simulink model "QueuingSys"  (R2019a)
settings: Solver=VariableStepAuto  StartTime=0.0  StopTime=100  RelTol=1e-3  EnableMultiTasking=on
undefined symbols (not defined in the file or in its folder): m, n
(part 4 of 5)

== system QueuingSys/Distro/MMPPArrivalTime57 ==
  MMPPArrivalTime : TriggerPort  TriggerType=function-call  IsSimulinkFunction=on  FunctionName=MMPPArrivalTime57  VariantControl=Variant
  Constant : Constant  Value=[0.495890558927082 0.224465538335651 0.279643902737266;0.534632777235722 0.436142153474273 0.0292250692900047;0.092615054756791 0.5282924947216 0.379092450521609]  SampleTime=-1
  D : Memory  InitialCondition=[0.615571878010216;0.243014654438024]  InheritSampleTime=on
  MMPP : MATLAB Function  TreatAsAtomicUnit=on
  Scope : Scope
  Scope1 : Scope
  T : Memory  InitialCondition=[0 0.156984443601208]  InheritSampleTime=on
  Uniform Random Number : UniformRandomNumber  Minimum=0  Seed=randi(5000)
  X : Memory  InitialCondition=2  InheritSampleTime=on
  t : ArgOut  DisableCoverage=on  ArgumentName=t
  wires:
  MMPP/5(lambda) -> Scope1/1
  D/1 -> MMPP/3("D ")
  MMPP/3(D) -> D/1
  Uniform Random Number/1 -> MMPP/5(rn)
  Constant/1 -> MMPP/4(M)
  MMPP/1(x) -> X/1
  MMPP/4(t) -> Scope/1, t/1
  MMPP/2(T) -> T/1
  T/1 -> MMPP/2("T ")
  X/1 -> MMPP/1("x ")

== system QueuingSys/Distro/MMPPArrivalTime58 ==
  MMPPArrivalTime : TriggerPort  TriggerType=function-call  IsSimulinkFunction=on  FunctionName=MMPPArrivalTime58  VariantControl=Variant
  Constant : Constant  Value=[0.117464299599952 0.152250567651033 0.121837267495483 0.159738037776046 0.149409502151923 0.125667086953631 0.173633238371933;0.148836709986002 0.0654920343032583 0.211732490033451 0.0881549893916536 0.208284652862022 0.1607543990228 0.116744724400813;0.197470470038891 0.0885266634647723 0.271156507153938 0.0722093849692539 0.0815411153869947 0.0614322791512611 0.227663579834889;0.1864274555943 0.0103838777427165 0.409677435278208 0.122348195829911 0.0518869784402073 0.187281746714561 0.0319943104000951;0.126572465826877 0.141130417950956 0.0378088808905448 0.0689503315505311 0.0237192420773743 0.137680845625693 0.464137816078024;0.175039845353253 0.101735916497746 0.151094631354237 0.0556980729938636 0.0793353789695721 0.239650762795073 0.197445392036255;0.164973290584489 0.169364680581661 0.0117698334218001 0.217271387849719 0.171379794259574 0.197448646262573 0.0677923670401836]  SampleTime=-1
  D : Memory  InitialCondition=[0.478618395085393;0.871374928352472]  InheritSampleTime=on
  MMPP : MATLAB Function  TreatAsAtomicUnit=on
  Scope : Scope
  Scope1 : Scope
  T : Memory  InitialCondition=[0 1.559364915483]  InheritSampleTime=on
  Uniform Random Number : UniformRandomNumber  Minimum=0  Seed=randi(5000)
  X : Memory  InitialCondition=6  InheritSampleTime=on
  t : ArgOut  DisableCoverage=on  ArgumentName=t
  wires:
  MMPP/5(lambda) -> Scope1/1
  D/1 -> MMPP/3("D ")
  MMPP/3(D) -> D/1
  Uniform Random Number/1 -> MMPP/5(rn)
  Constant/1 -> MMPP/4(M)
  MMPP/1(x) -> X/1
  MMPP/4(t) -> Scope/1, t/1
  MMPP/2(T) -> T/1
  T/1 -> MMPP/2("T ")
  X/1 -> MMPP/1("x ")

== system QueuingSys/Distro/MMPPArrivalTime59 ==
  MMPPArrivalTime : TriggerPort  TriggerType=function-call  IsSimulinkFunction=on  FunctionName=MMPPArrivalTime59  VariantControl=Variant
  Constant : Constant  Value=[0.231262783024567 0.402791363012738 0.0948533617147688 0.271092492247926;0.0697184986098729 0.168350419424436 0.447863652650022 0.314067429315669;0.290718579095752 0.248549728531608 0.221419645417609 0.23931204695503;0.198727445571336 0.024332155822817 0.395134296999519 0.381806101606328]  SampleTime=-1
  D : Memory  InitialCondition=[0.855831450381452;0.683244278757409]  InheritSampleTime=on
  MMPP : MATLAB Function  TreatAsAtomicUnit=on
  Scope : Scope
  Scope1 : Scope
  T : Memory  InitialCondition=[0 0.710690788050334]  InheritSampleTime=on
  Uniform Random Number : UniformRandomNumber  Minimum=0  Seed=randi(5000)
  X : Memory  InitialCondition=4  InheritSampleTime=on
  t : ArgOut  DisableCoverage=on  ArgumentName=t
  wires:
  MMPP/5(lambda) -> Scope1/1
  D/1 -> MMPP/3("D ")
  MMPP/3(D) -> D/1
  Uniform Random Number/1 -> MMPP/5(rn)
  Constant/1 -> MMPP/4(M)
  MMPP/1(x) -> X/1
  MMPP/4(t) -> Scope/1, t/1
  MMPP/2(T) -> T/1
  T/1 -> MMPP/2("T ")
  X/1 -> MMPP/1("x ")

== system QueuingSys/Distro/MMPPArrivalTime6 ==
  MMPPArrivalTime : TriggerPort  TriggerType=function-call  IsSimulinkFunction=on  FunctionName=MMPPArrivalTime6  VariantControl=Variant
  Constant : Constant  Value=[0.250507598802563 0.00575836632236452 0.241732742346078 0.106524945827142 0.0546304957988412 0.0757771957326207 0.00306838001227584 0.262000275158114;0.213829098700513 0.0821489794411499 0.0291299514633987 0.0513785838767398 0.144072248886932 0.221128259764545 0.0801765496174517 0.178136328249269;0.176775975083446 0.192228796343153 0.0437597869569795 0.0432089637665705 0.156678771137183 0.198701035186719 0.121669517073395 0.0669771544525552;0.152925028273588 0.130491673688067 0.17811334512996 0.15072607663695 0.0370775567647717 0.174721475639328 0.0436770439629412 0.132267799904395;0.0243848532441192 0.198795339726575 0.0820689931976927 0.135013541705003 0.211462701380172 0.113200342586652 0.0386322211834196 0.196442006976368;0.142385390519024 0.118197861166519 0.000436315012846692 0.053916013505201 0.131905377599712 0.0309585826029522 0.211431829922112 0.310768629671633;0.142032133138769 0.191920306557968 0.0833867878121167 0.202441621995813 0.0122590319747366 0.0624359393591409 0.123589953751878 0.181934225409577;0.0186792993654353 0.173625228000155 0.103940916450372 0.0182519190268161 0.218892903050549 0.174709111656949 0.179111063379142 0.112789559070582]  SampleTime=-1
  D : Memory  InitialCondition=[0.939412832737864;0.668081838726903]  InheritSampleTime=on
  MMPP : MATLAB Function  TreatAsAtomicUnit=on
  Scope : Scope
  Scope1 : Scope
  T : Memory  InitialCondition=[0 1.06872364839379]  InheritSampleTime=on
  Uniform Random Number : UniformRandomNumber  Minimum=0  Seed=randi(5000)
  X : Memory  InitialCondition=6  InheritSampleTime=on
  t : ArgOut  DisableCoverage=on  ArgumentName=t
  wires:
  MMPP/5(lambda) -> Scope1/1
  D/1 -> MMPP/3("D ")
  MMPP/3(D) -> D/1
  Uniform Random Number/1 -> MMPP/5(rn)
  Constant/1 -> MMPP/4(M)
  MMPP/1(x) -> X/1
  MMPP/4(t) -> Scope/1, t/1
  MMPP/2(T) -> T/1
  T/1 -> MMPP/2("T ")
  X/1 -> MMPP/1("x ")

== system QueuingSys/Distro/MMPPArrivalTime60 ==
  MMPPArrivalTime : TriggerPort  TriggerType=function-call  IsSimulinkFunction=on  FunctionName=MMPPArrivalTime60  VariantControl=Variant
  Constant : Constant  Value=[0.251439420992681 0.282465734529176 0.21753405163543 0.248560792842713;0.413879197984796 0.374781847180622 0.105519995757237 0.105818959077344;0.303504570548581 0.299042275864003 0.14904088149141 0.248412272096006;0.267232062980786 0.0879037163277221 0.298586996365245 0.346277224326246]  SampleTime=-1
  D : Memory  InitialCondition=[0.971466220988457;0.142859491474701]  InheritSampleTime=on
  MMPP : MATLAB Function  TreatAsAtomicUnit=on
  Scope : Scope
  Scope1 : Scope
  T : Memory  InitialCondition=[0 0.100773601526713]  InheritSampleTime=on
  Uniform Random Number : UniformRandomNumber  Minimum=0  Seed=randi(5000)
  X : Memory  InitialCondition=4  InheritSampleTime=on
  t : ArgOut  DisableCoverage=on  ArgumentName=t
  wires:
  MMPP/5(lambda) -> Scope1/1
  D/1 -> MMPP/3("D ")
  MMPP/3(D) -> D/1
  Uniform Random Number/1 -> MMPP/5(rn)
  Constant/1 -> MMPP/4(M)
  MMPP/1(x) -> X/1
  MMPP/4(t) -> Scope/1, t/1
  MMPP/2(T) -> T/1
  T/1 -> MMPP/2("T ")
  X/1 -> MMPP/1("x ")

== system QueuingSys/Distro/MMPPArrivalTime61 ==
  MMPPArrivalTime : TriggerPort  TriggerType=function-call  IsSimulinkFunction=on  FunctionName=MMPPArrivalTime61  VariantControl=Variant
  Constant : Constant  Value=[0.0358658607429067 0.260359110359736 0.148116048686889 0.0322610841777047 0.194713547529203 0.210107210579012 0.118577137924549;0.0937133367239626 0.384413016622962 0.110342319234354 0.0592148433271614 0.0235130452159556 0.304154682419081 0.0246487564565236;0.222979157181099 0.16066326660415 0.226310679066277 0.173302451037125 0.0589131279285746 0.132076418659366 0.0257548995234086;0.234150624710435 0.242815220932874 0.216523830357875 0.086173211946885 0.119390073926354 0.00659370497323011 0.0943533331523461;0.00188538259517628 0.0926285684260663 0.160587593259976 0.153080009834936 0.222787394842429 0.241763525746582 0.127267525294835;0.0784162169784009 0.072486403944959 0.230510152685508 0.246964485470099 0.173356981929177 0.0772016178102217 0.121064141181634;0.194340193386068 0.181098035578836 0.085018577843058 0.233610039249951 0.0182113629890858 0.287181029427603 0.00054076152539777]  SampleTime=-1
  D : Memory  InitialCondition=[0.345075963786048;0.656386819847764]  InheritSampleTime=on
  MMPP : MATLAB Function  TreatAsAtomicUnit=on
  Scope : Scope
  Scope1 : Scope
  T : Memory  InitialCondition=[0 0.985768972397712]  InheritSampleTime=on
  Uniform Random Number : UniformRandomNumber  Minimum=0  Seed=randi(5000)
  X : Memory  InitialCondition=6  InheritSampleTime=on
  t : ArgOut  DisableCoverage=on  ArgumentName=t
  wires:
  MMPP/5(lambda) -> Scope1/1
  D/1 -> MMPP/3("D ")
  MMPP/3(D) -> D/1
  Uniform Random Number/1 -> MMPP/5(rn)
  Constant/1 -> MMPP/4(M)
  MMPP/1(x) -> X/1
  MMPP/4(t) -> Scope/1, t/1
  MMPP/2(T) -> T/1
  T/1 -> MMPP/2("T ")
  X/1 -> MMPP/1("x ")

== system QueuingSys/Distro/MMPPArrivalTime62 ==
  MMPPArrivalTime : TriggerPort  TriggerType=function-call  IsSimulinkFunction=on  FunctionName=MMPPArrivalTime62  VariantControl=Variant
  Constant : Constant  Value=[0.247308267794237 0.266096721471469 0.486595010734294;0.331732714707182 0.470092222229744 0.198175063063074;0.0786618557616189 0.702310692833433 0.219027451404948]  SampleTime=-1
  D : Memory  InitialCondition=[0.764782048395018;0.396143550272663]  InheritSampleTime=on
  MMPP : MATLAB Function  TreatAsAtomicUnit=on
  Scope : Scope
  Scope1 : Scope
  T : Memory  InitialCondition=[0 0.37967184174422]  InheritSampleTime=on
  Uniform Random Number : UniformRandomNumber  Minimum=0  Seed=randi(5000)
  X : Memory  InitialCondition=1  InheritSampleTime=on
  t : ArgOut  DisableCoverage=on  ArgumentName=t
  wires:
  MMPP/5(lambda) -> Scope1/1
  D/1 -> MMPP/3("D ")
  MMPP/3(D) -> D/1
  Uniform Random Number/1 -> MMPP/5(rn)
  Constant/1 -> MMPP/4(M)
  MMPP/1(x) -> X/1
  MMPP/4(t) -> Scope/1, t/1
  MMPP/2(T) -> T/1
  T/1 -> MMPP/2("T ")
  X/1 -> MMPP/1("x ")

== system QueuingSys/Distro/MMPPArrivalTime63 ==
  MMPPArrivalTime : TriggerPort  TriggerType=function-call  IsSimulinkFunction=on  FunctionName=MMPPArrivalTime63  VariantControl=Variant
  Constant : Constant  Value=[0.166928932561933 0.055803987024089 0.109082674494602 0.0179486702325859 0.02153650878461 0.308306792921275 0.320392433980906;0.316629515146962 0.0254701410861867 0.241644244401003 0.0491344715849214 0.191286096910339 0.00834379500220388 0.167491735868384;0.194453066390585 0.169920474521602 0.104466983598958 0.11161823124551 0.190106682215482 0.0389266299213377 0.190507932106525;0.0786959675674802 0.137596414508794 0.104326289371514 0.229672454088435 0.0894776055535089 0.214020763911083 0.146210504999185;0.250619427316203 0.157930641553448 0.0875680364579376 0.108908184003506 0.12122772956099 0.00446419732290429 0.269281783785012;0.256491647078896 0.237826507391034 0.174415613949228 0.0848829850073848 0.0124632359493631 0.140064868260182 0.0938551423639124;0.112705456997265 0.0801367732819646 0.296086178328367 0.0237037121439084 0.143337905840896 0.304619408797618 0.039410564609981]  SampleTime=-1
  D : Memory  InitialCondition=[0.741751248827562;0.396930610524544]  InheritSampleTime=on
  MMPP : MATLAB Function  TreatAsAtomicUnit=on
  Scope : Scope
  Scope1 : Scope
  T : Memory  InitialCondition=[0 0.444415362208905]  InheritSampleTime=on
  Uniform Random Number : UniformRandomNumber  Minimum=0  Seed=randi(5000)
  X : Memory  InitialCondition=5  InheritSampleTime=on
  t : ArgOut  DisableCoverage=on  ArgumentName=t
  wires:
  MMPP/5(lambda) -> Scope1/1
  D/1 -> MMPP/3("D ")
  MMPP/3(D) -> D/1
  Uniform Random Number/1 -> MMPP/5(rn)
  Constant/1 -> MMPP/4(M)
  MMPP/1(x) -> X/1
  MMPP/4(t) -> Scope/1, t/1
  MMPP/2(T) -> T/1
  T/1 -> MMPP/2("T ")
  X/1 -> MMPP/1("x ")

== system QueuingSys/Distro/MMPPArrivalTime64 ==
  MMPPArrivalTime : TriggerPort  TriggerType=function-call  IsSimulinkFunction=on  FunctionName=MMPPArrivalTime64  VariantControl=Variant
  Constant : Constant  Value=[0.253372852603573 0.20919113420105 0.121021072669466 0.416414940525911;0.0559145655595751 0.0881784103349402 0.445706447082528 0.410200577022956;0.257294137861287 0.0579182221477352 0.238294449612016 0.446493190378962;0.140920190325539 0.495188586238886 0.0121105593146895 0.351780664120886]  SampleTime=-1
  D : Memory  InitialCondition=[0.241524416499248;0.117559394450335]  InheritSampleTime=on
  MMPP : MATLAB Function  TreatAsAtomicUnit=on
  Scope : Scope
  Scope1 : Scope
  T : Memory  InitialCondition=[0 0.0810687700939244]  InheritSampleTime=on
  Uniform Random Number : UniformRandomNumber  Minimum=0  Seed=randi(5000)
  X : Memory  InitialCondition=4  InheritSampleTime=on
  t : ArgOut  DisableCoverage=on  ArgumentName=t
  wires:
  MMPP/5(lambda) -> Scope1/1
  D/1 -> MMPP/3("D ")
  MMPP/3(D) -> D/1
  Uniform Random Number/1 -> MMPP/5(rn)
  Constant/1 -> MMPP/4(M)
  MMPP/1(x) -> X/1
  MMPP/4(t) -> Scope/1, t/1
  MMPP/2(T) -> T/1
  T/1 -> MMPP/2("T ")
  X/1 -> MMPP/1("x ")

== system QueuingSys/Distro/MMPPArrivalTime65 ==
  MMPPArrivalTime : TriggerPort  TriggerType=function-call  IsSimulinkFunction=on  FunctionName=MMPPArrivalTime65  VariantControl=Variant
  Constant : Constant  Value=[0.549844630973916 0.338847708387615 0.111307660638468;0.333556942042834 0.447189164535601 0.219253893421565;0.10006016282948 0.773222811159549 0.126717026010971]  SampleTime=-1
  D : Memory  InitialCondition=[0.748681324956193;0.206451980537833]  InheritSampleTime=on
  MMPP : MATLAB Function  TreatAsAtomicUnit=on
  Scope : Scope
  Scope1 : Scope
  T : Memory  InitialCondition=[0 0.201939024525195]  InheritSampleTime=on
  Uniform Random Number : UniformRandomNumber  Minimum=0  Seed=randi(5000)
  X : Memory  InitialCondition=3  InheritSampleTime=on
  t : ArgOut  DisableCoverage=on  ArgumentName=t
  wires:
  MMPP/5(lambda) -> Scope1/1
  D/1 -> MMPP/3("D ")
  MMPP/3(D) -> D/1
  Uniform Random Number/1 -> MMPP/5(rn)
  Constant/1 -> MMPP/4(M)
  MMPP/1(x) -> X/1
  MMPP/4(t) -> Scope/1, t/1
  MMPP/2(T) -> T/1
  T/1 -> MMPP/2("T ")
  X/1 -> MMPP/1("x ")

== system QueuingSys/Distro/MMPPArrivalTime66 ==
  MMPPArrivalTime : TriggerPort  TriggerType=function-call  IsSimulinkFunction=on  FunctionName=MMPPArrivalTime66  VariantControl=Variant
  Constant : Constant  Value=[0.174897441669732 0.0424927776052225 0.0445045068663381 0.220321246736531 0.275050785461624 0.242733241660553;0.131554523259652 0.158420549423664 0.223653701579918 0.185745756595696 0.233328605252044 0.0672968638890254;0.227621062434643 0.199314720826553 0.0480715904558601 0.160621004218325 0.170212962490831 0.194158659573788;0.198719948275677 0.206199630682328 0.206074496316485 0.129996364112708 0.196214546663832 0.0627950139489701;0.353858190340985 0.204554481526254 0.0571139797351515 0.126975169791725 0.0393806539666986 0.218117524639185;0.125294306566581 0.150011410169528 0.179705469986616 0.295159725415406 0.159314552720421 0.0905145351414476]  SampleTime=-1
  D : Memory  InitialCondition=[0.92794993715419;0.0301212458382484]  InheritSampleTime=on
  MMPP : MATLAB Function  TreatAsAtomicUnit=on
  Scope : Scope
  Scope1 : Scope
  T : Memory  InitialCondition=[0 0.0291139793409204]  InheritSampleTime=on
  Uniform Random Number : UniformRandomNumber  Minimum=0  Seed=randi(5000)
  X : Memory  InitialCondition=3  InheritSampleTime=on
  t : ArgOut  DisableCoverage=on  ArgumentName=t
  wires:
  MMPP/5(lambda) -> Scope1/1
  D/1 -> MMPP/3("D ")
  MMPP/3(D) -> D/1
  Uniform Random Number/1 -> MMPP/5(rn)
  Constant/1 -> MMPP/4(M)
  MMPP/1(x) -> X/1
  MMPP/4(t) -> Scope/1, t/1
  MMPP/2(T) -> T/1
  T/1 -> MMPP/2("T ")
  X/1 -> MMPP/1("x ")

== system QueuingSys/Distro/MMPPArrivalTime67 ==
  MMPPArrivalTime : TriggerPort  TriggerType=function-call  IsSimulinkFunction=on  FunctionName=MMPPArrivalTime67  VariantControl=Variant
  Constant : Constant  Value=[0.0425556968497329 0.200251093881359 0.187273814877379 0.122274467720345 0.114624778705721 0.209172761607279 0.123847386358184;0.044741241176505 0.155519347030819 0.148248369113252 0.181287484173783 0.209837691770696 0.237018449365303 0.0233474173696413;0.240085680029991 0.106660943232373 0.235685771482993 0.211790886426931 0.168407643119897 0.0306895343501551 0.0066795413576602;0.0722072549032886 0.176739221636763 0.201276525895344 0.129646447267744 0.181390693657606 0.041816113081434 0.196923743557821;0.0778430763117883 0.0882774920468442 0.0157849692749159 0.38550356272757 0.298514846582343 0.0567538302489661 0.077322222807573;0.171892309969137 0.182477577733946 0.162605629848858 0.011742234275033 0.121317245667039 0.165895505284285 0.184069497221702;0.19273805198627 0.197132274919083 0.158110847144895 0.0933832362683892 0.210351901399878 0.0915051160735984 0.0567785722078853]  SampleTime=-1
  D : Memory  InitialCondition=[0.672555516137938;0.084327464233755]  InheritSampleTime=on
  MMPP : MATLAB Function  TreatAsAtomicUnit=on
  Scope : Scope
  Scope1 : Scope
  T : Memory  InitialCondition=[0 0.0843474651761423]  InheritSampleTime=on
  Uniform Random Number : UniformRandomNumber  Minimum=0  Seed=randi(5000)
  X : Memory  InitialCondition=1  InheritSampleTime=on
  t : ArgOut  DisableCoverage=on  ArgumentName=t
  wires:
  MMPP/5(lambda) -> Scope1/1
  D/1 -> MMPP/3("D ")
  MMPP/3(D) -> D/1
  Uniform Random Number/1 -> MMPP/5(rn)
  Constant/1 -> MMPP/4(M)
  MMPP/1(x) -> X/1
  MMPP/4(t) -> Scope/1, t/1
  MMPP/2(T) -> T/1
  T/1 -> MMPP/2("T ")
  X/1 -> MMPP/1("x ")

== system QueuingSys/Distro/MMPPArrivalTime68 ==
  MMPPArrivalTime : TriggerPort  TriggerType=function-call  IsSimulinkFunction=on  FunctionName=MMPPArrivalTime68  VariantControl=Variant
  Constant : Constant  Value=[0.355381651643604 0.644618348356396;0.58088111081965 0.41911888918035]  SampleTime=-1
  D : Memory  InitialCondition=[0.00494271342247377;0.352234711999676]  InheritSampleTime=on
  MMPP : MATLAB Function  TreatAsAtomicUnit=on
  Scope : Scope
  Scope1 : Scope
  T : Memory  InitialCondition=[0 0.252234179692325]  InheritSampleTime=on
  Uniform Random Number : UniformRandomNumber  Minimum=0  Seed=randi(5000)
  X : Memory  InitialCondition=2  InheritSampleTime=on
  t : ArgOut  DisableCoverage=on  ArgumentName=t
  wires:
  MMPP/5(lambda) -> Scope1/1
  D/1 -> MMPP/3("D ")
  MMPP/3(D) -> D/1
  Uniform Random Number/1 -> MMPP/5(rn)
  Constant/1 -> MMPP/4(M)
  MMPP/1(x) -> X/1
  MMPP/4(t) -> Scope/1, t/1
  MMPP/2(T) -> T/1
  T/1 -> MMPP/2("T ")
  X/1 -> MMPP/1("x ")

== system QueuingSys/Distro/MMPPArrivalTime69 ==
  MMPPArrivalTime : TriggerPort  TriggerType=function-call  IsSimulinkFunction=on  FunctionName=MMPPArrivalTime69  VariantControl=Variant
  Constant : Constant  Value=[0.168210140073948 0.00963497680894319 0.0870622047727576 0.336060152651297 0.399032525693054;0.219407157087732 0.00718184263548427 0.282678391368939 0.234658747156754 0.256073861751091;0.0790346860561059 0.27834696130578 0.185672784282632 0.271928325514253 0.185017242841229;0.202020052898992 0.0117448926256568 0.445134979318637 0.228341196518164 0.11275887863855;0.0751979882779372 0.299241765706561 0.117079746243966 0.306630728915269 0.201849770856267]  SampleTime=-1
  D : Memory  InitialCondition=[0.875941509519679;0.473321817886645]  InheritSampleTime=on
  MMPP : MATLAB Function  TreatAsAtomicUnit=on
  Scope : Scope
  Scope1 : Scope
  T : Memory  InitialCondition=[0 0.494761062055696]  InheritSampleTime=on
  Uniform Random Number : UniformRandomNumber  Minimum=0  Seed=randi(5000)
  X : Memory  InitialCondition=4  InheritSampleTime=on
  t : ArgOut  DisableCoverage=on  ArgumentName=t
  wires:
  MMPP/5(lambda) -> Scope1/1
  D/1 -> MMPP/3("D ")
  MMPP/3(D) -> D/1
  Uniform Random Number/1 -> MMPP/5(rn)
  Constant/1 -> MMPP/4(M)
  MMPP/1(x) -> X/1
  MMPP/4(t) -> Scope/1, t/1
  MMPP/2(T) -> T/1
  T/1 -> MMPP/2("T ")
  X/1 -> MMPP/1("x ")

== system QueuingSys/Distro/MMPPArrivalTime7 ==
  MMPPArrivalTime : TriggerPort  TriggerType=function-call  IsSimulinkFunction=on  FunctionName=MMPPArrivalTime7  VariantControl=Variant
  Constant : Constant  Value=[0.00440429574457922 0.246422563961028 0.340480223800199 0.294699348164565 0.113993568329629;0.128190909138978 0.063847459455475 0.186519810212613 0.334426224821765 0.287015596371169;0.366399400715378 0.230000921703626 0.0797290507439633 0.292453731280117 0.0314168955569165;0.189405588130297 0.190686730440017 0.0912504594069354 0.19294163405858 0.335715587964171;0.269668605010426 0.246725024561676 0.0941429195137778 0.0491615106032638 0.340301940310856]  SampleTime=-1
  D : Memory  InitialCondition=[0.575207697512688;0.766517273968399]  InheritSampleTime=on
  MMPP : MATLAB Function  TreatAsAtomicUnit=on
  Scope : Scope
  Scope1 : Scope
  T : Memory  InitialCondition=[0 0.959627924197696]  InheritSampleTime=on
  Uniform Random Number : UniformRandomNumber  Minimum=0  Seed=randi(5000)
  X : Memory  InitialCondition=5  InheritSampleTime=on
  t : ArgOut  DisableCoverage=on  ArgumentName=t
  wires:
  MMPP/5(lambda) -> Scope1/1
  D/1 -> MMPP/3("D ")
  MMPP/3(D) -> D/1
  Uniform Random Number/1 -> MMPP/5(rn)
  Constant/1 -> MMPP/4(M)
  MMPP/1(x) -> X/1
  MMPP/4(t) -> Scope/1, t/1
  MMPP/2(T) -> T/1
  T/1 -> MMPP/2("T ")
  X/1 -> MMPP/1("x ")

== system QueuingSys/Distro/MMPPArrivalTime70 ==
  MMPPArrivalTime : TriggerPort  TriggerType=function-call  IsSimulinkFunction=on  FunctionName=MMPPArrivalTime70  VariantControl=Variant
  Constant : Constant  Value=[0.184875017423423 0.251834301521587 0.070422688566232 0.0487552977955828 0.161399737097333 0.214674977483829 0.0680379801120133;0.029454419391542 0.268437825133967 0.0541946430833975 0.1681715216119 0.130827444427254 0.106588293837232 0.242325852514707;0.174981772581958 0.0412083785599854 0.0453644967316862 0.211839361391622 0.202807184215442 0.0863422773566494 0.237456529162657;0.266449790061194 0.0521116500649548 0.266803107822909 0.0537979076785723 0.0156003937452723 0.199088915759373 0.146148234867725;0.000185459135012 0.0387636445938314 0.237467768114476 0.242793221076715 0.278107486481083 0.148243701509911 0.054438719088971;0.0294694268520089 0.175222644888175 0.179928432815074 0.255578329211691 0.160297188532769 0.0515935417161645 0.147910435984119;0.116901080656893 0.13000129658975 0.207763603853018 0.079068254777043 0.13555064010877 0.0171366669656287 0.313578457048897]  SampleTime=-1
  D : Memory  InitialCondition=[0.96602377253342;0.929880550051944]  InheritSampleTime=on
  MMPP : MATLAB Function  TreatAsAtomicUnit=on
  Scope : Scope
  Scope1 : Scope
  T : Memory  InitialCondition=[0 2.52044238537079]  InheritSampleTime=on
  Uniform Random Number : UniformRandomNumber  Minimum=0  Seed=randi(5000)
  X : Memory  InitialCondition=6  InheritSampleTime=on
  t : ArgOut  DisableCoverage=on  ArgumentName=t
  wires:
  MMPP/5(lambda) -> Scope1/1
  D/1 -> MMPP/3("D ")
  MMPP/3(D) -> D/1
  Uniform Random Number/1 -> MMPP/5(rn)
  Constant/1 -> MMPP/4(M)
  MMPP/1(x) -> X/1
  MMPP/4(t) -> Scope/1, t/1
  MMPP/2(T) -> T/1
  T/1 -> MMPP/2("T ")
  X/1 -> MMPP/1("x ")

== system QueuingSys/Distro/MMPPArrivalTime8 ==
  MMPPArrivalTime : TriggerPort  TriggerType=function-call  IsSimulinkFunction=on  FunctionName=MMPPArrivalTime8  VariantControl=Variant
  Constant : Constant  Value=[0.00541948361554863 0.0718633374864293 0.0335026305008963 0.25664860449536 0.362548723792226 0.161008190114829 0.109009029994712;0.188688202412436 0.21031355746448 0.161366589270669 0.0217408680501493 0.192189535520082 0.219695632636304 0.00600561464587938;0.103703335914736 0.0657090455826601 0.156276003579455 0.100593680317048 0.199447862801747 0.178132987451184 0.196137084353171;0.123353607680428 0.129997259854191 0.0950926617949369 0.200846578107168 0.110125154690635 0.123721579506277 0.216863158366364;0.223660483226027 0.221826313066034 0.0918448888170575 0.142732851619665 0.0568284024068118 0.199446110522334 0.0636609503420706;0.24379361284987 0.1026719510418 0.204734113819026 0.0394064050593579 0.189690574981947 0.0810380126758198 0.138665329572178;0.242102851003073 0.103357887259098 0.238974725454145 0.0668129223225235 0.0861908089991003 0.0708435794794879 0.191717225482572]  SampleTime=-1
  D : Memory  InitialCondition=[0.2185834125899;0.722665277239192]  InheritSampleTime=on
  MMPP : MATLAB Function  TreatAsAtomicUnit=on
  Scope : Scope
  Scope1 : Scope
  T : Memory  InitialCondition=[0 1.0821014357494]  InheritSampleTime=on
  Uniform Random Number : UniformRandomNumber  Minimum=0  Seed=randi(5000)
  X : Memory  InitialCondition=3  InheritSampleTime=on
  t : ArgOut  DisableCoverage=on  ArgumentName=t
  wires:
  MMPP/5(lambda) -> Scope1/1
  D/1 -> MMPP/3("D ")
  MMPP/3(D) -> D/1
  Uniform Random Number/1 -> MMPP/5(rn)
  Constant/1 -> MMPP/4(M)
  MMPP/1(x) -> X/1
  MMPP/4(t) -> Scope/1, t/1
  MMPP/2(T) -> T/1
  T/1 -> MMPP/2("T ")
  X/1 -> MMPP/1("x ")

== system QueuingSys/Distro/MMPPArrivalTime9 ==
  MMPPArrivalTime : TriggerPort  TriggerType=function-call  IsSimulinkFunction=on  FunctionName=MMPPArrivalTime9  VariantControl=Variant
  Constant : Constant  Value=[0.0375076099316973 0.136557313810652 0.137423751655545 0.16375841632861 0.16147002980198 0.178008303053219 0.185274575418297;0.150344660652943 0.100683300622566 0.20128743469548 0.180534980346273 0.189196458619877 0.0388692713592656 0.139083893703595;0.296261636207599 0.0349689844713893 0.0201397930385374 0.194062188113362 0.308815927264416 0.0111887798340739 0.134562691070623;0.102725381411523 0.0313538495881027 0.0850780113671224 0.143557434603251 0.272169915990176 0.2137980569974 0.151317350042425;0.149223044352787 0.0252040138961668 0.221868248711811 0.220254774991551 0.214595784209209 0.126268758270724 0.0425853755677511;0.302789553354404 0.151698156986724 0.00352736819655097 0.252258996349342 0.0964784885361964 0.11283488245285 0.0804125541239324;0.154149400894005 0.299668075901612 0.0535685917323428 0.223775966144629 0.0187125804643076 0.184559806015341 0.065565578847763]  SampleTime=-1
  D : Memory  InitialCondition=[0.942632406182967;0.641570357548248]  InheritSampleTime=on
  MMPP : MATLAB Function  TreatAsAtomicUnit=on
  Scope : Scope
  Scope1 : Scope
  T : Memory  InitialCondition=[0 0.922719522129056]  InheritSampleTime=on
  Uniform Random Number : UniformRandomNumber  Minimum=0  Seed=randi(5000)
  X : Memory  InitialCondition=2  InheritSampleTime=on
  t : ArgOut  DisableCoverage=on  ArgumentName=t
  wires:
  MMPP/5(lambda) -> Scope1/1
  D/1 -> MMPP/3("D ")
  MMPP/3(D) -> D/1
  Uniform Random Number/1 -> MMPP/5(rn)
  Constant/1 -> MMPP/4(M)
  MMPP/1(x) -> X/1
  MMPP/4(t) -> Scope/1, t/1
  MMPP/2(T) -> T/1
  T/1 -> MMPP/2("T ")
  X/1 -> MMPP/1("x ")

== matlab function QueuingSys/Distro/MMPPArrivalTime2/MMPP ==
  data: x input; T input; D input; x output; M input; T output; D output; t output; rn input; lambda output
function [x,T,D,t,lambda] = fcn(x,T,D,M,rn)
lambda = sum(M(x,:))-M(x,x);
trn = expinv(rn,lambda);
if trn > T(2)
    D =rand(2,1);
    T2 = expinv(D(2),lambda);
    j = 1;
    a = 0;
    b = sum(M(x,1:j));
    while ~(a < D(1) < b)
        j = j +1;
        a = sum(M(x,1:j));
        b = sum(M(x,1:j));
    end
    x = j;
    T(1) = T(2);
    T(2) = T2;
    lambda = sum(M(x,:))-M(x,x);
    trn = expinv(rn,lambda);
end
% x = j;
t = trn;% x(end);

== matlab function QueuingSys/Distro/MMPPArrivalTime1/MMPP ==
  data: x input; T input; D input; x output; M input; T output; D output; t output; rn input; lambda output
function [x,T,D,t,lambda] = fcn(x,T,D,M,rn)
lambda = sum(M(x,:))-M(x,x);
trn = expinv(rn,lambda);
if trn > T(2)
    D =rand(2,1);
    T2 = expinv(D(2),lambda);
    j = 1;
    a = 0;
    b = sum(M(x,1:j));
    while ~(a < D(1) < b)
        j = j +1;
        a = sum(M(x,1:j));
        b = sum(M(x,1:j));
    end
    x = j;
    T(1) = T(2);
    T(2) = T2;
    lambda = sum(M(x,:))-M(x,x);
    trn = expinv(rn,lambda);
end
% x = j;
t = trn;% x(end);

== matlab function QueuingSys/Distro/MMPPArrivalTime3/MMPP ==
  data: x input; T input; D input; x output; M input; T output; D output; t output; rn input; lambda output
function [x,T,D,t,lambda] = fcn(x,T,D,M,rn)
lambda = sum(M(x,:))-M(x,x);
trn = expinv(rn,lambda);
if trn > T(2)
    D =rand(2,1);
    T2 = expinv(D(2),lambda);
    j = 1;
    a = 0;
    b = sum(M(x,1:j));
    while ~(a < D(1) < b)
        j = j +1;
        a = sum(M(x,1:j));
        b = sum(M(x,1:j));
    end
    x = j;
    T(1) = T(2);
    T(2) = T2;
    lambda = sum(M(x,:))-M(x,x);
    trn = expinv(rn,lambda);
end
% x = j;
t = trn;% x(end);

== matlab function QueuingSys/Distro/MMPPArrivalTime4/MMPP ==
  data: x input; T input; D input; x output; M input; T output; D output; t output; rn input; lambda output
function [x,T,D,t,lambda] = fcn(x,T,D,M,rn)
lambda = sum(M(x,:))-M(x,x);
trn = expinv(rn,lambda);
if trn > T(2)
    D =rand(2,1);
    T2 = expinv(D(2),lambda);
    j = 1;
    a = 0;
    b = sum(M(x,1:j));
    while ~(a < D(1) < b)
        j = j +1;
        a = sum(M(x,1:j));
        b = sum(M(x,1:j));
    end
    x = j;
    T(1) = T(2);
    T(2) = T2;
    lambda = sum(M(x,:))-M(x,x);
    trn = expinv(rn,lambda);
end
% x = j;
t = trn;% x(end);

== matlab function QueuingSys/Distro/MMPPArrivalTime5/MMPP ==
  data: x input; T input; D input; x output; M input; T output; D output; t output; rn input; lambda output
function [x,T,D,t,lambda] = fcn(x,T,D,M,rn)
lambda = sum(M(x,:))-M(x,x);
trn = expinv(rn,lambda);
if trn > T(2)
    D =rand(2,1);
    T2 = expinv(D(2),lambda);
    j = 1;
    a = 0;
    b = sum(M(x,1:j));
    while ~(a < D(1) < b)
        j = j +1;
        a = sum(M(x,1:j));
        b = sum(M(x,1:j));
    end
    x = j;
    T(1) = T(2);
    T(2) = T2;
    lambda = sum(M(x,:))-M(x,x);
    trn = expinv(rn,lambda);
end
% x = j;
t = trn;% x(end);

== matlab function QueuingSys/Distro/MMPPArrivalTime6/MMPP ==
  data: x input; T input; D input; x output; M input; T output; D output; t output; rn input; lambda output
function [x,T,D,t,lambda] = fcn(x,T,D,M,rn)
lambda = sum(M(x,:))-M(x,x);
trn = expinv(rn,lambda);
if trn > T(2)
    D =rand(2,1);
    T2 = expinv(D(2),lambda);
    j = 1;
    a = 0;
    b = sum(M(x,1:j));
    while ~(a < D(1) < b)
        j = j +1;
        a = sum(M(x,1:j));
        b = sum(M(x,1:j));
    end
    x = j;
    T(1) = T(2);
    T(2) = T2;
    lambda = sum(M(x,:))-M(x,x);
    trn = expinv(rn,lambda);
end
% x = j;
t = trn;% x(end);

== matlab function QueuingSys/Distro/MMPPArrivalTime7/MMPP ==
  data: x input; T input; D input; x output; M input; T output; D output; t output; rn input; lambda output
function [x,T,D,t,lambda] = fcn(x,T,D,M,rn)
lambda = sum(M(x,:))-M(x,x);
trn = expinv(rn,lambda);
if trn > T(2)
    D =rand(2,1);
    T2 = expinv(D(2),lambda);
    j = 1;
    a = 0;
    b = sum(M(x,1:j));
    while ~(a < D(1) < b)
        j = j +1;
        a = sum(M(x,1:j));
        b = sum(M(x,1:j));
    end
    x = j;
    T(1) = T(2);
    T(2) = T2;
    lambda = sum(M(x,:))-M(x,x);
    trn = expinv(rn,lambda);
end
% x = j;
t = trn;% x(end);

== matlab function QueuingSys/Distro/MMPPArrivalTime8/MMPP ==
  data: x input; T input; D input; x output; M input; T output; D output; t output; rn input; lambda output
function [x,T,D,t,lambda] = fcn(x,T,D,M,rn)
lambda = sum(M(x,:))-M(x,x);
trn = expinv(rn,lambda);
if trn > T(2)
    D =rand(2,1);
    T2 = expinv(D(2),lambda);
    j = 1;
    a = 0;
    b = sum(M(x,1:j));
    while ~(a < D(1) < b)
        j = j +1;
        a = sum(M(x,1:j));
        b = sum(M(x,1:j));
    end
    x = j;
    T(1) = T(2);
    T(2) = T2;
    lambda = sum(M(x,:))-M(x,x);
    trn = expinv(rn,lambda);
end
% x = j;
t = trn;% x(end);

== matlab function QueuingSys/MATLAB Function ==
  data: cap1 input; stop output; cap2 input; Pn input
function stop  = fcn(cap1,cap2,Pn)
max1 = 4;
max2= 3;
stop = 0;
if Pn == 1
    if cap1 == max1
        stop = 1;
    end
end
if Pn == 2
    if cap2 == max2
        stop = 1;
    end
end
% if cap1 == max1 && e(1) == 0 && e(2) == 0
%     e(1) = 1;
%     T(1) = time;
% elseif cap1 == max1 && e(2) == 1 && e(1) == 0
%     stop = 1;
%     T(1) = time;
% end
% if cap2 == max2 && e(2) == 0 && e(1) == 0
%     e(2) = 1;
%     T(2) = time;
% elseif cap2 == max2 && e(1) == 1 && e(2) == 0
%     stop = 1;
%     T(2) = time;
% 
% end

end

== matlab function QueuingSys/Distro/MMPPArrivalTime9/MMPP ==
  data: x input; T input; D input; x output; M input; T output; D output; t output; rn input; lambda output
function [x,T,D,t,lambda] = fcn(x,T,D,M,rn)
lambda = sum(M(x,:))-M(x,x);
trn = expinv(rn,lambda);
if trn > T(2)
    D =rand(2,1);
    T2 = expinv(D(2),lambda);
    j = 1;
    a = 0;
    b = sum(M(x,1:j));
    while ~(a < D(1) < b)
        j = j +1;
        a = sum(M(x,1:j));
        b = sum(M(x,1:j));
    end
    x = j;
    T(1) = T(2);
    T(2) = T2;
    lambda = sum(M(x,:))-M(x,x);
    trn = expinv(rn,lambda);
end
% x = j;
t = trn;% x(end);

== matlab function QueuingSys/Distro/MMPPArrivalTime10/MMPP ==
  data: x input; T input; D input; x output; M input; T output; D output; t output; rn input; lambda output
function [x,T,D,t,lambda] = fcn(x,T,D,M,rn)
lambda = sum(M(x,:))-M(x,x);
trn = expinv(rn,lambda);
if trn > T(2)
    D =rand(2,1);
    T2 = expinv(D(2),lambda);
    j = 1;
    a = 0;
    b = sum(M(x,1:j));
    while ~(a < D(1) < b)
        j = j +1;
        a = sum(M(x,1:j));
        b = sum(M(x,1:j));
    end
    x = j;
    T(1) = T(2);
    T(2) = T2;
    lambda = sum(M(x,:))-M(x,x);
    trn = expinv(rn,lambda);
end
% x = j;
t = trn;% x(end);

== matlab function QueuingSys/Distro/MMPPArrivalTime11/MMPP ==
  data: x input; T input; D input; x output; M input; T output; D output; t output; rn input; lambda output
function [x,T,D,t,lambda] = fcn(x,T,D,M,rn)
lambda = sum(M(x,:))-M(x,x);
trn = expinv(rn,lambda);
if trn > T(2)
    D =rand(2,1);
    T2 = expinv(D(2),lambda);
    j = 1;
    a = 0;
    b = sum(M(x,1:j));
    while ~(a < D(1) < b)
        j = j +1;
        a = sum(M(x,1:j));
        b = sum(M(x,1:j));
    end
    x = j;
    T(1) = T(2);
    T(2) = T2;
    lambda = sum(M(x,:))-M(x,x);
    trn = expinv(rn,lambda);
end
% x = j;
t = trn;% x(end);

== matlab function QueuingSys/Distro/MMPPArrivalTime12/MMPP ==
  data: x input; T input; D input; x output; M input; T output; D output; t output; rn input; lambda output
function [x,T,D,t,lambda] = fcn(x,T,D,M,rn)
lambda = sum(M(x,:))-M(x,x);
trn = expinv(rn,lambda);
if trn > T(2)
    D =rand(2,1);
    T2 = expinv(D(2),lambda);
    j = 1;
    a = 0;
    b = sum(M(x,1:j));
    while ~(a < D(1) < b)
        j = j +1;
        a = sum(M(x,1:j));
        b = sum(M(x,1:j));
    end
    x = j;
    T(1) = T(2);
    T(2) = T2;
    lambda = sum(M(x,:))-M(x,x);
    trn = expinv(rn,lambda);
end
% x = j;
t = trn;% x(end);

== matlab function QueuingSys/Distro/MMPPArrivalTime13/MMPP ==
  data: x input; T input; D input; x output; M input; T output; D output; t output; rn input; lambda output
function [x,T,D,t,lambda] = fcn(x,T,D,M,rn)
lambda = sum(M(x,:))-M(x,x);
trn = expinv(rn,lambda);
if trn > T(2)
    D =rand(2,1);
    T2 = expinv(D(2),lambda);
    j = 1;
    a = 0;
    b = sum(M(x,1:j));
    while ~(a < D(1) < b)
        j = j +1;
        a = sum(M(x,1:j));
        b = sum(M(x,1:j));
    end
    x = j;
    T(1) = T(2);
    T(2) = T2;
    lambda = sum(M(x,:))-M(x,x);
    trn = expinv(rn,lambda);
end
% x = j;
t = trn;% x(end);

== matlab function QueuingSys/Distro/MMPPArrivalTime14/MMPP ==
  data: x input; T input; D input; x output; M input; T output; D output; t output; rn input; lambda output
function [x,T,D,t,lambda] = fcn(x,T,D,M,rn)
lambda = sum(M(x,:))-M(x,x);
trn = expinv(rn,lambda);
if trn > T(2)
    D =rand(2,1);
    T2 = expinv(D(2),lambda);
    j = 1;
    a = 0;
    b = sum(M(x,1:j));
    while ~(a < D(1) < b)
        j = j +1;
        a = sum(M(x,1:j));
        b = sum(M(x,1:j));
    end
    x = j;
    T(1) = T(2);
    T(2) = T2;
    lambda = sum(M(x,:))-M(x,x);
    trn = expinv(rn,lambda);
end
% x = j;
t = trn;% x(end);

== matlab function QueuingSys/Distro/MMPPArrivalTime15/MMPP ==
  data: x input; T input; D input; x output; M input; T output; D output; t output; rn input; lambda output
function [x,T,D,t,lambda] = fcn(x,T,D,M,rn)
lambda = sum(M(x,:))-M(x,x);
trn = expinv(rn,lambda);
if trn > T(2)
    D =rand(2,1);
    T2 = expinv(D(2),lambda);
    j = 1;
    a = 0;
    b = sum(M(x,1:j));
    while ~(a < D(1) < b)
        j = j +1;
        a = sum(M(x,1:j));
        b = sum(M(x,1:j));
    end
    x = j;
    T(1) = T(2);
    T(2) = T2;
    lambda = sum(M(x,:))-M(x,x);
    trn = expinv(rn,lambda);
end
% x = j;
t = trn;% x(end);

== matlab function QueuingSys/Distro/MMPPArrivalTime16/MMPP ==
  data: x input; T input; D input; x output; M input; T output; D output; t output; rn input; lambda output
function [x,T,D,t,lambda] = fcn(x,T,D,M,rn)
lambda = sum(M(x,:))-M(x,x);
trn = expinv(rn,lambda);
if trn > T(2)
    D =rand(2,1);
    T2 = expinv(D(2),lambda);
    j = 1;
    a = 0;
    b = sum(M(x,1:j));
    while ~(a < D(1) < b)
        j = j +1;
        a = sum(M(x,1:j));
        b = sum(M(x,1:j));
    end
    x = j;
    T(1) = T(2);
    T(2) = T2;
    lambda = sum(M(x,:))-M(x,x);
    trn = expinv(rn,lambda);
end
% x = j;
t = trn;% x(end);

== matlab function QueuingSys/Distro/MMPPArrivalTime17/MMPP ==
  data: x input; T input; D input; x output; M input; T output; D output; t output; rn input; lambda output
function [x,T,D,t,lambda] = fcn(x,T,D,M,rn)
lambda = sum(M(x,:))-M(x,x);
trn = expinv(rn,lambda);
if trn > T(2)
    D =rand(2,1);
    T2 = expinv(D(2),lambda);
    j = 1;
    a = 0;
    b = sum(M(x,1:j));
    while ~(a < D(1) < b)
        j = j +1;
        a = sum(M(x,1:j));
        b = sum(M(x,1:j));
    end
    x = j;
    T(1) = T(2);
    T(2) = T2;
    lambda = sum(M(x,:))-M(x,x);
    trn = expinv(rn,lambda);
end
% x = j;
t = trn;% x(end);

== matlab function QueuingSys/Distro/MMPPArrivalTime18/MMPP ==
  data: x input; T input; D input; x output; M input; T output; D output; t output; rn input; lambda output
function [x,T,D,t,lambda] = fcn(x,T,D,M,rn)
lambda = sum(M(x,:))-M(x,x);
trn = expinv(rn,lambda);
if trn > T(2)
    D =rand(2,1);
    T2 = expinv(D(2),lambda);
    j = 1;
    a = 0;
    b = sum(M(x,1:j));
    while ~(a < D(1) < b)
        j = j +1;
        a = sum(M(x,1:j));
        b = sum(M(x,1:j));
    end
    x = j;
    T(1) = T(2);
    T(2) = T2;
    lambda = sum(M(x,:))-M(x,x);
    trn = expinv(rn,lambda);
end
% x = j;
t = trn;% x(end);

== matlab function QueuingSys/Distro/MMPPArrivalTime19/MMPP ==
  data: x input; T input; D input; x output; M input; T output; D output; t output; rn input; lambda output
function [x,T,D,t,lambda] = fcn(x,T,D,M,rn)
lambda = sum(M(x,:))-M(x,x);
trn = expinv(rn,lambda);
if trn > T(2)
    D =rand(2,1);
    T2 = expinv(D(2),lambda);
    j = 1;
    a = 0;
    b = sum(M(x,1:j));
    while ~(a < D(1) < b)
        j = j +1;
        a = sum(M(x,1:j));
        b = sum(M(x,1:j));
    end
    x = j;
    T(1) = T(2);
    T(2) = T2;
    lambda = sum(M(x,:))-M(x,x);
    trn = expinv(rn,lambda);
end
% x = j;
t = trn;% x(end);

== matlab function QueuingSys/Distro/MMPPArrivalTime20/MMPP ==
  data: x input; T input; D input; x output; M input; T output; D output; t output; rn input; lambda output
function [x,T,D,t,lambda] = fcn(x,T,D,M,rn)
lambda = sum(M(x,:))-M(x,x);
trn = expinv(rn,lambda);
if trn > T(2)
    D =rand(2,1);
    T2 = expinv(D(2),lambda);
    j = 1;
    a = 0;
    b = sum(M(x,1:j));
    while ~(a < D(1) < b)
        j = j +1;
        a = sum(M(x,1:j));
        b = sum(M(x,1:j));
    end
    x = j;
    T(1) = T(2);
    T(2) = T2;
    lambda = sum(M(x,:))-M(x,x);
    trn = expinv(rn,lambda);
end
% x = j;
t = trn;% x(end);

== matlab function QueuingSys/Distro/MMPPArrivalTime21/MMPP ==
  data: x input; T input; D input; x output; M input; T output; D output; t output; rn input; lambda output
function [x,T,D,t,lambda] = fcn(x,T,D,M,rn)
lambda = sum(M(x,:))-M(x,x);
trn = expinv(rn,lambda);
if trn > T(2)
    D =rand(2,1);
    T2 = expinv(D(2),lambda);
    j = 1;
    a = 0;
    b = sum(M(x,1:j));
    while ~(a < D(1) < b)
        j = j +1;
        a = sum(M(x,1:j));
        b = sum(M(x,1:j));
    end
    x = j;
    T(1) = T(2);
    T(2) = T2;
    lambda = sum(M(x,:))-M(x,x);
    trn = expinv(rn,lambda);
end
% x = j;
t = trn;% x(end);

== matlab function QueuingSys/Distro/MMPPArrivalTime22/MMPP ==
  data: x input; T input; D input; x output; M input; T output; D output; t output; rn input; lambda output
function [x,T,D,t,lambda] = fcn(x,T,D,M,rn)
lambda = sum(M(x,:))-M(x,x);
trn = expinv(rn,lambda);
if trn > T(2)
    D =rand(2,1);
    T2 = expinv(D(2),lambda);
    j = 1;
    a = 0;
    b = sum(M(x,1:j));
    while ~(a < D(1) < b)
        j = j +1;
        a = sum(M(x,1:j));
        b = sum(M(x,1:j));
    end
    x = j;
    T(1) = T(2);
    T(2) = T2;
    lambda = sum(M(x,:))-M(x,x);
    trn = expinv(rn,lambda);
end
% x = j;
t = trn;% x(end);

== matlab function QueuingSys/Distro/MMPPArrivalTime23/MMPP ==
  data: x input; T input; D input; x output; M input; T output; D output; t output; rn input; lambda output
function [x,T,D,t,lambda] = fcn(x,T,D,M,rn)
lambda = sum(M(x,:))-M(x,x);
trn = expinv(rn,lambda);
if trn > T(2)
    D =rand(2,1);
    T2 = expinv(D(2),lambda);
    j = 1;
    a = 0;
    b = sum(M(x,1:j));
    while ~(a < D(1) < b)
        j = j +1;
        a = sum(M(x,1:j));
        b = sum(M(x,1:j));
    end
    x = j;
    T(1) = T(2);
    T(2) = T2;
    lambda = sum(M(x,:))-M(x,x);
    trn = expinv(rn,lambda);
end
% x = j;
t = trn;% x(end);

== matlab function QueuingSys/Distro/MMPPArrivalTime24/MMPP ==
  data: x input; T input; D input; x output; M input; T output; D output; t output; rn input; lambda output
function [x,T,D,t,lambda] = fcn(x,T,D,M,rn)
lambda = sum(M(x,:))-M(x,x);
trn = expinv(rn,lambda);
if trn > T(2)
    D =rand(2,1);
    T2 = expinv(D(2),lambda);
    j = 1;
    a = 0;
    b = sum(M(x,1:j));
    while ~(a < D(1) < b)
        j = j +1;
        a = sum(M(x,1:j));
        b = sum(M(x,1:j));
    end
    x = j;
    T(1) = T(2);
    T(2) = T2;
    lambda = sum(M(x,:))-M(x,x);
    trn = expinv(rn,lambda);
end
% x = j;
t = trn;% x(end);

== matlab function QueuingSys/Distro/MMPPArrivalTime25/MMPP ==
  data: x input; T input; D input; x output; M input; T output; D output; t output; rn input; lambda output
function [x,T,D,t,lambda] = fcn(x,T,D,M,rn)
lambda = sum(M(x,:))-M(x,x);
trn = expinv(rn,lambda);
if trn > T(2)
    D =rand(2,1);
    T2 = expinv(D(2),lambda);
    j = 1;
    a = 0;
    b = sum(M(x,1:j));
    while ~(a < D(1) < b)
        j = j +1;
        a = sum(M(x,1:j));
        b = sum(M(x,1:j));
    end
    x = j;
    T(1) = T(2);
    T(2) = T2;
    lambda = sum(M(x,:))-M(x,x);
    trn = expinv(rn,lambda);
end
% x = j;
t = trn;% x(end);

== matlab function QueuingSys/Distro/MMPPArrivalTime26/MMPP ==
  data: x input; T input; D input; x output; M input; T output; D output; t output; rn input; lambda output
function [x,T,D,t,lambda] = fcn(x,T,D,M,rn)
lambda = sum(M(x,:))-M(x,x);
trn = expinv(rn,lambda);
if trn > T(2)
    D =rand(2,1);
    T2 = expinv(D(2),lambda);
    j = 1;
    a = 0;
    b = sum(M(x,1:j));
    while ~(a < D(1) < b)
        j = j +1;
        a = sum(M(x,1:j));
        b = sum(M(x,1:j));
    end
    x = j;
    T(1) = T(2);
    T(2) = T2;
    lambda = sum(M(x,:))-M(x,x);
    trn = expinv(rn,lambda);
end
% x = j;
t = trn;% x(end);

== matlab function QueuingSys/Distro/MMPPArrivalTime27/MMPP ==
  data: x input; T input; D input; x output; M input; T output; D output; t output; rn input; lambda output
function [x,T,D,t,lambda] = fcn(x,T,D,M,rn)
lambda = sum(M(x,:))-M(x,x);
trn = expinv(rn,lambda);
if trn > T(2)
    D =rand(2,1);
    T2 = expinv(D(2),lambda);
    j = 1;
    a = 0;
    b = sum(M(x,1:j));
    while ~(a < D(1) < b)
        j = j +1;
        a = sum(M(x,1:j));
        b = sum(M(x,1:j));
    end
    x = j;
    T(1) = T(2);
    T(2) = T2;
    lambda = sum(M(x,:))-M(x,x);
    trn = expinv(rn,lambda);
end
% x = j;
t = trn;% x(end);

== matlab function QueuingSys/Distro/MMPPArrivalTime28/MMPP ==
  data: x input; T input; D input; x output; M input; T output; D output; t output; rn input; lambda output
function [x,T,D,t,lambda] = fcn(x,T,D,M,rn)
lambda = sum(M(x,:))-M(x,x);
trn = expinv(rn,lambda);
if trn > T(2)
    D =rand(2,1);
    T2 = expinv(D(2),lambda);
    j = 1;
    a = 0;
    b = sum(M(x,1:j));
    while ~(a < D(1) < b)
        j = j +1;
        a = sum(M(x,1:j));
        b = sum(M(x,1:j));
    end
    x = j;
    T(1) = T(2);
    T(2) = T2;
    lambda = sum(M(x,:))-M(x,x);
    trn = expinv(rn,lambda);
end
% x = j;
t = trn;% x(end);

== matlab function QueuingSys/Distro/MMPPArrivalTime29/MMPP ==
  data: x input; T input; D input; x output; M input; T output; D output; t output; rn input; lambda output
function [x,T,D,t,lambda] = fcn(x,T,D,M,rn)
lambda = sum(M(x,:))-M(x,x);
trn = expinv(rn,lambda);
if trn > T(2)
    D =rand(2,1);
    T2 = expinv(D(2),lambda);
    j = 1;
    a = 0;
    b = sum(M(x,1:j));
    while ~(a < D(1) < b)
        j = j +1;
        a = sum(M(x,1:j));
        b = sum(M(x,1:j));
    end
    x = j;
    T(1) = T(2);
    T(2) = T2;
    lambda = sum(M(x,:))-M(x,x);
    trn = expinv(rn,lambda);
end
% x = j;
t = trn;% x(end);

== matlab function QueuingSys/Distro/MMPPArrivalTime30/MMPP ==
  data: x input; T input; D input; x output; M input; T output; D output; t output; rn input; lambda output
function [x,T,D,t,lambda] = fcn(x,T,D,M,rn)
lambda = sum(M(x,:))-M(x,x);
trn = expinv(rn,lambda);
if trn > T(2)
    D =rand(2,1);
    T2 = expinv(D(2),lambda);
    j = 1;
    a = 0;
    b = sum(M(x,1:j));
    while ~(a < D(1) < b)
        j = j +1;
        a = sum(M(x,1:j));
        b = sum(M(x,1:j));
    end
    x = j;
    T(1) = T(2);
    T(2) = T2;
    lambda = sum(M(x,:))-M(x,x);
    trn = expinv(rn,lambda);
end
% x = j;
t = trn;% x(end);

== matlab function QueuingSys/Distro/MMPPArrivalTime31/MMPP ==
  data: x input; T input; D input; x output; M input; T output; D output; t output; rn input; lambda output
function [x,T,D,t,lambda] = fcn(x,T,D,M,rn)
lambda = sum(M(x,:))-M(x,x);
trn = expinv(rn,lambda);
if trn > T(2)
    D =rand(2,1);
    T2 = expinv(D(2),lambda);
    j = 1;
    a = 0;
    b = sum(M(x,1:j));
    while ~(a < D(1) < b)
        j = j +1;
        a = sum(M(x,1:j));
        b = sum(M(x,1:j));
    end
    x = j;
    T(1) = T(2);
    T(2) = T2;
    lambda = sum(M(x,:))-M(x,x);
    trn = expinv(rn,lambda);
end
% x = j;
t = trn;% x(end);

== matlab function QueuingSys/Distro/MMPPArrivalTime32/MMPP ==
  data: x input; T input; D input; x output; M input; T output; D output; t output; rn input; lambda output
function [x,T,D,t,lambda] = fcn(x,T,D,M,rn)
lambda = sum(M(x,:))-M(x,x);
trn = expinv(rn,lambda);
if trn > T(2)
    D =rand(2,1);
    T2 = expinv(D(2),lambda);
    j = 1;
    a = 0;
    b = sum(M(x,1:j));
    while ~(a < D(1) < b)
        j = j +1;
        a = sum(M(x,1:j));
        b = sum(M(x,1:j));
    end
    x = j;
    T(1) = T(2);
    T(2) = T2;
    lambda = sum(M(x,:))-M(x,x);
    trn = expinv(rn,lambda);
end
% x = j;
t = trn;% x(end);

== matlab function QueuingSys/Distro/MMPPArrivalTime33/MMPP ==
  data: x input; T input; D input; x output; M input; T output; D output; t output; rn input; lambda output
function [x,T,D,t,lambda] = fcn(x,T,D,M,rn)
lambda = sum(M(x,:))-M(x,x);
trn = expinv(rn,lambda);
if trn > T(2)
    D =rand(2,1);
    T2 = expinv(D(2),lambda);
    j = 1;
    a = 0;
    b = sum(M(x,1:j));
    while ~(a < D(1) < b)
        j = j +1;
        a = sum(M(x,1:j));
        b = sum(M(x,1:j));
    end
    x = j;
    T(1) = T(2);
    T(2) = T2;
    lambda = sum(M(x,:))-M(x,x);
    trn = expinv(rn,lambda);
end
% x = j;
t = trn;% x(end);

== matlab function QueuingSys/Distro/MMPPArrivalTime34/MMPP ==
  data: x input; T input; D input; x output; M input; T output; D output; t output; rn input; lambda output
function [x,T,D,t,lambda] = fcn(x,T,D,M,rn)
lambda = sum(M(x,:))-M(x,x);
trn = expinv(rn,lambda);
if trn > T(2)
    D =rand(2,1);
    T2 = expinv(D(2),lambda);
    j = 1;
    a = 0;
    b = sum(M(x,1:j));
    while ~(a < D(1) < b)
        j = j +1;
        a = sum(M(x,1:j));
        b = sum(M(x,1:j));
    end
    x = j;
    T(1) = T(2);
    T(2) = T2;
    lambda = sum(M(x,:))-M(x,x);
    trn = expinv(rn,lambda);
end
% x = j;
t = trn;% x(end);

== matlab function QueuingSys/Distro/MMPPArrivalTime35/MMPP ==
  data: x input; T input; D input; x output; M input; T output; D output; t output; rn input; lambda output
function [x,T,D,t,lambda] = fcn(x,T,D,M,rn)
lambda = sum(M(x,:))-M(x,x);
trn = expinv(rn,lambda);
if trn > T(2)
    D =rand(2,1);
    T2 = expinv(D(2),lambda);
    j = 1;
    a = 0;
    b = sum(M(x,1:j));
    while ~(a < D(1) < b)
        j = j +1;
        a = sum(M(x,1:j));
        b = sum(M(x,1:j));
    end
    x = j;
    T(1) = T(2);
    T(2) = T2;
    lambda = sum(M(x,:))-M(x,x);
    trn = expinv(rn,lambda);
end
% x = j;
t = trn;% x(end);
